simulink subsystem "simulation_pause_subsystem"  (R2021b)
settings: Solver=VariableStepAuto  StartTime=0.0  StopTime=10.0  RelTol=1e-3
settings Model: Creator=Whitney  LastModifiedBy=whitney

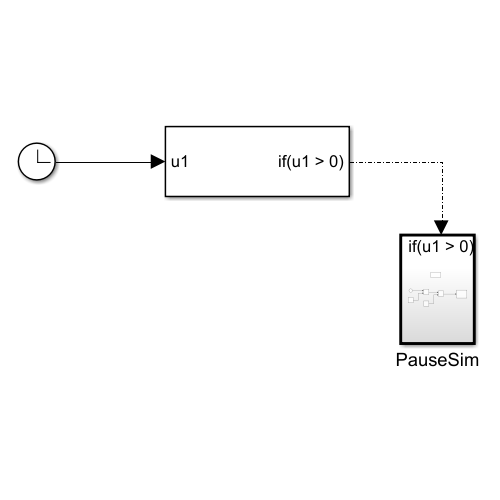
[thumbnail: Simulink's stored preview of the top-level diagram]
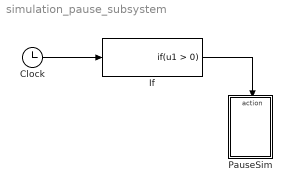
== system simulation_pause_subsystem ==
  Clock : Clock
  If : If  ShowElse=off
  PauseSim : Subsystem
  wires:
  If/1 -> PauseSim/Action
  Clock/1 -> If/1

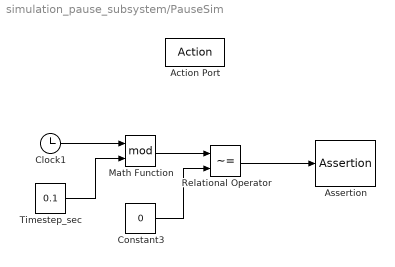
== system simulation_pause_subsystem/PauseSim ==
  Action Port : ActionPort
  Assertion : Assertion  AssertionFailFcn=|  StopWhenAssertionFail=off
      | set_param(bdroot,'SimulationCommand','pause'),
      | disp(sprintf('\nSimulation paused.')), isPaused = true
  Clock1 : Clock
  Constant3 : Constant  Value=0
  Math Function : Math  Operator=mod  SaturateOnIntegerOverflow=on
  Relational Operator : RelationalOperator  Operator=~=  OutDataTypeStr=boolean  RndMeth=Nearest
  Timestep_sec : Constant  Value=0.1
  wires:
  Timestep_sec/1 -> Math Function/2
  Relational Operator/1 -> Assertion/1
  Constant3/1 -> Relational Operator/2
  Math Function/1 -> Relational Operator/1
  Clock1/1 -> Math Function/1
